simulink model "BuckBoost_ideal"  (R2015b)
settings: Solver=VariableStepAuto  StartTime=0.0  StopTime=0.01  RelTol=0.001
values from neighbouring files (symbols this model uses):
  Rload = 10    [BuckBoost_script.m]
libraries: fl_lib x7, elec_lib x5, nesl_utility x5
settings Model: Creator=lukaskiechle  LastModifiedBy=lukaskiechle
settings DebuggingCC: MaxConsecutiveZCsMsg=none
settings SimscapeCC: SimscapeLogType=all  SimscapeLogOpenViewer=on

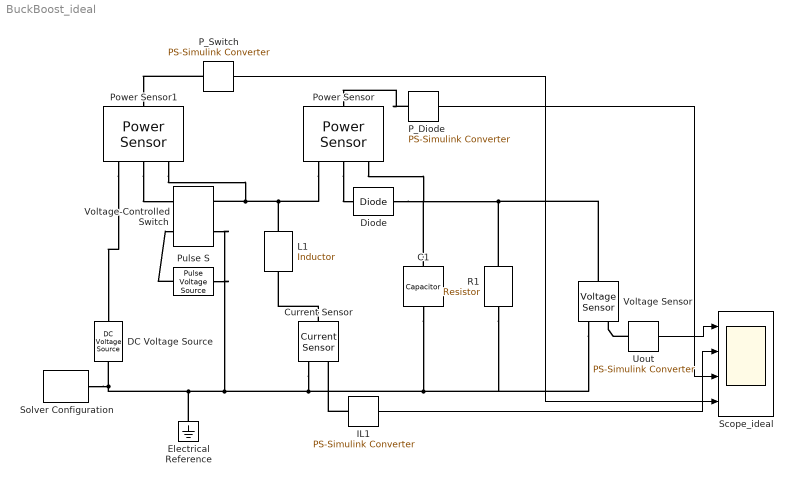
== system BuckBoost_ideal ==
  C1 : fl_lib/Electrical/Electrical Elements/Capacitor  c=C1 F  r=1e-9 Ohm  g=0 1/Ohm  i_specify=off  i_priority=None  i=0 A  v_specify=off  v_priority=None  v=0 V  vc_specify=off  vc_priority=None  vc=0 V
  Current Sensor : fl_lib/Electrical/Electrical Sensors/Current Sensor
  DC Voltage Source : fl_lib/Electrical/Electrical Sources/DC Voltage Source  v0=Uin V
  Diode : elec_lib/Semiconductor Devices/Diode  ModelType=1  Vf=UF V  Ron=1E-6 Ohm  Goff=1E-9 S  Rz=0.1 Ohm  Vz=160 V  C_PWL=0 F  prmExp=2  I12=[ 0.0137 0.545 ] A  V12=[ 0.6 0.7 ] V  I1=0.0137 A  V1=0.6 V  RS=0.01 Ohm  IS=1e-12 A  Tmeas=25 C  ec=1  BV=Inf V  C_param=1  CJ0=5 pF  VJ=1 V  Mgrad=0.5  Vvec=[ 0.1 10 100 ] V  Cvec=[ 3.5 1 0.4 ] pF  FC=0.5  Q_param=1  Irrm=-7.15 A  iF=4 A  didt=-750 A/us  trr=115 ns  TT=50 ns  tau=100 ns  T_param=1  IS_T2=1.25e-7 A  I1_T2=0.245 A  V1_T2=0.5 V  Tmeas2=125 C  EG_param=1  EG=1.11 eV  XTI_param=1  XTI=3  dBVdT=0 V/K  Tdevice=25 C  Rth=[ 0 10 ] K/W  thermal_mass_parameterization=1  thermal_mass=[ 0 1 ] J/K  thermal_time_constant=[ 0 10 ] s  thermal_mass_initial_temperatures=[ 25 25 ] C
  Electrical Reference : fl_lib/Electrical/Electrical Elements/Electrical Reference
  IL1 : nesl_utility/PS-Simulink Converter  PhysicalDomain=network_engine_domain  SubClassName=ps_output  LeftPortType=input  RightPortType=output  PseudoPeriodic=off  Frequencies=[]  Unit=A  AffineConversion=off
  L1 : fl_lib/Electrical/Electrical Elements/Inductor  l=L1 H  r=0 Ohm  g=1e-9 1/Ohm  i_specify=off  i_priority=None  i=0 A  v_specify=off  v_priority=None  v=0 V  i_L_specify=off  i_L_priority=None  i_L=0 A
  P_Diode : nesl_utility/PS-Simulink Converter  PhysicalDomain=network_engine_domain  SubClassName=ps_output  LeftPortType=input  RightPortType=output  PseudoPeriodic=off  Frequencies=[]  Unit=W  AffineConversion=off
  P_Switch : nesl_utility/PS-Simulink Converter  PhysicalDomain=network_engine_domain  SubClassName=ps_output  LeftPortType=input  RightPortType=output  PseudoPeriodic=off  Frequencies=[]  Unit=W  AffineConversion=off
  Power Sensor : elec_lib/Sensors/Power Sensor  measurement_type=1  averaging_period=1 ms
  Power Sensor1 : elec_lib/Sensors/Power Sensor  measurement_type=1  averaging_period=1 ms
  Pulse S : elec_lib/Additional Components/SPICE-Compatible Components/Sources/Pulse Voltage Source  V1=0 V  V2=Upulse V  TD=0 s  TR=1e-9 s  TF=1e-9 s  PW=Ton s  PER=Twidth s
  R1 : fl_lib/Electrical/Electrical Elements/Resistor  R=Rload Ohm  i_specify=off  i_priority=None  i=0 A  v_specify=off  v_priority=None  v=0 V
  Scope_ideal : Scope  NumInputPorts=4
  Solver Configuration : nesl_utility/Solver Configuration  PhysicalDomain=network_engine_domain  SubClassName=solver  LeftPortType=input  RightPortType=generic  Accelerate=off  Tones=[]  Harmonics=[]  SimulateNoise=off  Profile=off  UseLocalSampling=off  EnableSwitchedLinearOptims=on  FrequencyDomain=off  UseCCode=off  RelTol=0.001  AbsTol=1e-06  MinStep=1e-09  ToWorkspace=off  RevertToSquareIcSolve=off  NumHomotopyIterations=100  PhasorMode=off  PhasorModeNumHarmonics=1  DoDC=on  ResidualTolerance=1e-09  UseLocalSolver=off  LocalSolverChoice=NE_BACKWARD_EULER_ADVANCER  LocalSolverSampleTime=0.001  DoFixedCost=off  MaxNonlinIter=3  MaxModeIter=2  LinearAlgebra=Sparse  DelaysMemoryBudget=1024  AutomaticFiltering=on  FilteringTimeConstant=0.001
  Uout : nesl_utility/PS-Simulink Converter  PhysicalDomain=network_engine_domain  SubClassName=ps_output  LeftPortType=input  RightPortType=output  PseudoPeriodic=off  Frequencies=[]  Unit=V  AffineConversion=off
  Voltage Sensor : fl_lib/Electrical/Electrical Sensors/Voltage Sensor
  Voltage-Controlled Switch : elec_lib/Additional Components/SPICE-Compatible Components/Passive Devices/Voltage-Controlled Switch  VT=Ut V  VH=Uh V  RON=1E-6 Ohm  ROFF=1E+9 Ohm  IC_state=-1
  wires:
  Uout/1 -> Scope_ideal/1
  IL1/1 -> Scope_ideal/2
  P_Diode/1 -> Scope_ideal/3
  P_Switch/1 -> Scope_ideal/4
  connections:
  Electrical Reference/LConn1 -- Voltage-Controlled Switch/RConn1 -- Pulse S/RConn1 -- R1/RConn1 -- Voltage Sensor/RConn2 -- C1/RConn1 -- Current Sensor/RConn2 -- Solver Configuration/RConn1 -- DC Voltage Source/RConn1
  Voltage Sensor/LConn1 -- Power Sensor/LConn3 -- Diode/LConn1 -- C1/LConn1 -- R1/LConn1
  Uout/LConn1 -- Voltage Sensor/RConn1
  Pulse S/LConn1 -- Voltage-Controlled Switch/LConn1
  Current Sensor/LConn1 -- L1/RConn1
  IL1/LConn1 -- Current Sensor/RConn1
  L1/LConn1 -- Power Sensor1/LConn3 -- Voltage-Controlled Switch/RConn2 -- Power Sensor/LConn1
  Power Sensor/LConn2 -- Diode/RConn1
  Power Sensor1/LConn1 -- DC Voltage Source/LConn1
  Power Sensor1/LConn2 -- Voltage-Controlled Switch/LConn2
  P_Switch/LConn1 -- Power Sensor1/RConn1
  P_Diode/LConn1 -- Power Sensor/RConn1
